simulink model "Mine_ROTPEN_nonlinear_unfinished"  (R2022b)
settings: Solver=ode23s  StartTime=0.0  StopTime=50  RelTol=1e-5  EnableMultiTasking=on
values from neighbouring files (symbols this model uses):
  B1 = 0.001    [Controled model.mat]
  B2 = 0.0001    [Controled model.mat]
  g = 9.81    [Controled model.mat]
  Jeq = 0.00018    [Controled model.mat]
  K = [98.2270291879 13.4441714398 -6.32469390722 -3.4975494389]    [Controled model.mat]
  Km = 0.0333    [Controled model.mat]
  Kt = 0.0333    [Controled model.mat]
  Lp = 0.153    [Controled model.mat]
  Mp = 0.027    [Controled model.mat]
  r = 0.0826    [Controled model.mat]
  Rm = 8.7    [Controled model.mat]
settings Model: Creator=p1318983x  LastModifiedBy=Mr Franklyn
settings SolverCC: AlgebraicLoopSolver=TrustRegion
settings DataIOCC: LimitDataPoints=on  SaveFormat=Array  SignalLoggingSaveFormat=ModelDataLogs  ReturnWorkspaceOutputs=off
settings OptimizationCC: ExpressionDepthLimit=2147483647  LifeSpan=inf
settings DebuggingCC: UnderspecifiedInitializationDetection=Classic  MergeDetectMultiDrivingBlocksExec=none  SolverPrmCheckMsg=warning  FcnCallInpInsideContextMsg=warning  UnconnectedInputMsg=warning  UnconnectedOutputMsg=warning  UnconnectedLineMsg=warning  StateNameClashWarn=warning  SFUnexpectedBacktrackingDiag=warning  SFNoUnconditionalDefaultTransitionDiag=warning  SFExecutionAtInitializationDiag=none  SFMachineParentedDataDiag=warning  ArithmeticOperatorsInVariantConditions=warning
settings HardwareCC: ProdBitPerPointer=32  ProdBitPerSizeT=32  ProdBitPerPtrDiffT=32  ProdLargestAtomicFloat=None  ProdIntDivRoundTo=Undefined  ProdEndianess=Unspecified  ProdWordSize=32  ProdHWDeviceType=32-bit Generic
settings ModelReferenceCC: EnableRefExpFcnMdlSchedulingChecks=on  PropagateSignalLabelsOutOfModel=off
settings SFSimCC: SimUseLocalCustomCode=off  CustomCodeUndefinedFunction=UseInterfaceOnly
settings RTWCC: RTWUseLocalCustomCode=off
settings CodeAppCC: StateflowObjectComments=on
settings GRTTargetCC: TargetLangStandard=C89/C90 (ANSI)  CombineOutputUpdateFcns=off  GRTInterface=on
settings ConfigComp: CovMetricSettings=dw  CovSaveCumulativeToWorkspaceVar=on  CovSaveSingleToWorkspaceVar=on  CovExternalEMLEnable=off

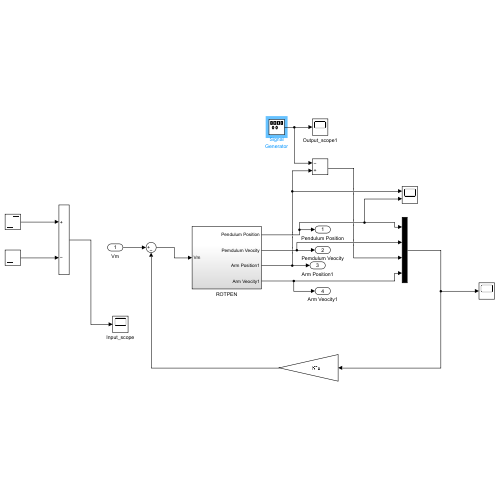
[thumbnail: Simulink's stored preview of the top-level diagram]
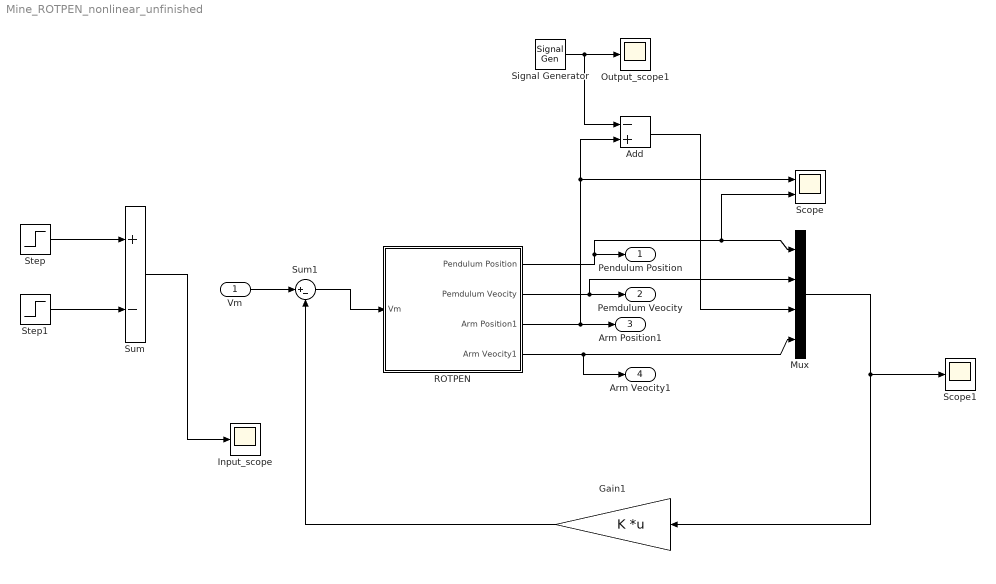
== system Mine_ROTPEN_nonlinear_unfinished ==
  Vm : Inport
  Add : Sum  Inputs=-+
  Gain1 : Gain  Gain=K  Multiplication=Matrix(K*u)
  Input_scope : Scope
  Mux : Mux
  Output_scope1 : Scope
  ROTPEN : Subsystem
  Scope : Scope  NumInputPorts=2
      settings: Tag=2
  Scope1 : Scope
  Signal Generator : SignalGenerator  WaveForm=square  Amplitude=0.2618  Frequency=0.05  Units=rad/sec
  Step : Step  Time=10  SampleTime=0
  Step1 : Step  Time=12  SampleTime=0
  Sum : Sum  Inputs=+-
  Sum1 : Sum  Inputs=|+-
  Pendulum Position : Outport
  Pemdulum Veocity : Outport  Port=2
  Arm Position1 : Outport  Port=3
  Arm Veocity1 : Outport  Port=4
  wires:
  Sum/1 -> Input_scope/1
  Mux/1 -> Scope1/1, Gain1/1
  Step/1 -> Sum/1
  Step1/1 -> Sum/2
  ROTPEN/1(Pendulum Position) -> Mux/1, Scope/2, Pendulum Position/1
  ROTPEN/2(Pemdulum Veocity) -> Mux/2, Pemdulum Veocity/1
  ROTPEN/3(Arm Position1) -> Add/2, Scope/1, Arm Position1/1
  Signal Generator/1 -> Add/1, Output_scope1/1
  ROTPEN/4(Arm Veocity1) -> Mux/4, Arm Veocity1/1
  Add/1 -> Mux/3
  Vm/1 -> Sum1/1
  Gain1/1 -> Sum1/2
  Sum1/1 -> ROTPEN/1(Vm)

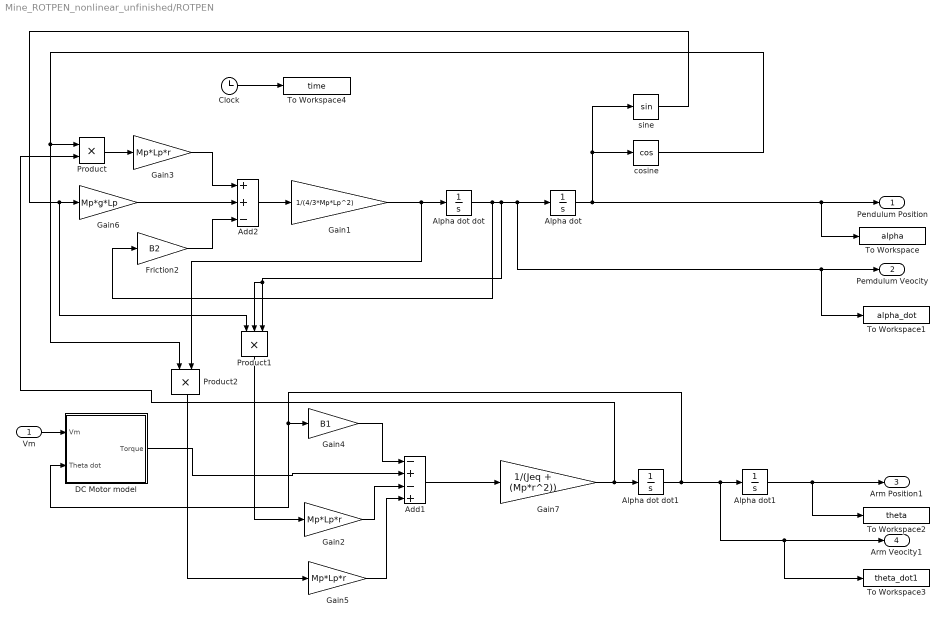
== system Mine_ROTPEN_nonlinear_unfinished/ROTPEN ==
  Vm : Inport
  Add1 : Sum  Inputs=-+-+
  Add2 : Sum  Inputs=++-
  Alpha dot : Integrator  InitialCondition=0.05
  Alpha dot dot : Integrator
  Alpha dot dot1 : Integrator
  Alpha dot1 : Integrator
  Clock : Clock
  DC Motor model : Subsystem
  Friction2 : Gain  Gain=B2
  Gain1 : Gain  Gain=1/(4/3*Mp*Lp^2)
  Gain2 : Gain  Gain=Mp*Lp*r
  Gain3 : Gain  Gain=Mp*Lp*r
  Gain4 : Gain  Gain=B1
  Gain5 : Gain  Gain=Mp*Lp*r
  Gain6 : Gain  Gain=Mp*g*Lp
  Gain7 : Gain  Gain=1/(Jeq + (Mp*r^2))
  Product : Product  RndMeth=Zero
  Product1 : Product  Inputs=3
  Product2 : Product
  To Workspace : ToWorkspace  VariableName=alpha  SampleTime=-1
  To Workspace1 : ToWorkspace  VariableName=alpha_dot  SampleTime=-1
  To Workspace2 : ToWorkspace  VariableName=theta  SampleTime=-1
  To Workspace3 : ToWorkspace  VariableName=theta_dot1  SampleTime=-1
  To Workspace4 : ToWorkspace  VariableName=time  SampleTime=-1
  cosine : Trigonometry  Operator=cos
  sine : Trigonometry
  Pendulum Position : Outport
  Pemdulum Veocity : Outport  Port=2
  Arm Position1 : Outport  Port=3
  Arm Veocity1 : Outport  Port=4
  wires:
  Alpha dot/1 -> sine/1, cosine/1, Pendulum Position/1, To Workspace/1
  sine/1 -> Product1/1, Gain6/1
  Add2/1 -> Gain1/1
  Product/1 -> Gain3/1
  Gain3/1 -> Add2/1
  Gain6/1 -> Add2/2
  Vm/1 -> DC Motor model/1(Vm)
  Friction2/1 -> Add2/3
  Clock/1 -> To Workspace4/1
  Gain2/1 -> Add1/3
  DC Motor model/1(Torque) -> Add1/2
  Gain4/1 -> Add1/1
  Gain5/1 -> Add1/4
  Alpha dot dot/1 -> Product1/2, Product1/3, Pemdulum Veocity/1, To Workspace1/1, Alpha dot/1, Friction2/1
  Product1/1 -> Gain2/1
  cosine/1 -> Product2/1, Product/1
  Product2/1 -> Gain5/1
  Gain1/1 -> Product2/2, Alpha dot dot/1
  Add1/1 -> Gain7/1
  Alpha dot dot1/1 -> DC Motor model/2(Theta dot), Gain4/1, To Workspace3/1, Arm Veocity1/1, Alpha dot1/1
  Alpha dot1/1 -> To Workspace2/1, Arm Position1/1
  Gain7/1 -> Alpha dot dot1/1, Product/2

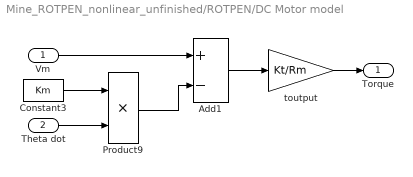
== system Mine_ROTPEN_nonlinear_unfinished/ROTPEN/DC Motor model ==
  Vm : Inport
  Theta dot : Inport  Port=2
  Add1 : Sum  Inputs=+-
  Constant3 : Constant  Value=Km
  Product9 : Product  RndMeth=Zero
  toutput : Gain  Gain=Kt/Rm
  Torque : Outport
  wires:
  Add1/1 -> toutput/1
  Constant3/1 -> Product9/1
  Product9/1 -> Add1/2
  Theta dot/1 -> Product9/2
  Vm/1 -> Add1/1
  toutput/1 -> Torque/1
